simulink model "es2_catena_aperta_1"  (R2014a)
settings: Solver=ode45  StartTime=0.0  StopTime=10.0  RelTol=1e-3
libraries: cstblocks x3
settings Model: Creator=HP  LastModifiedBy=HP

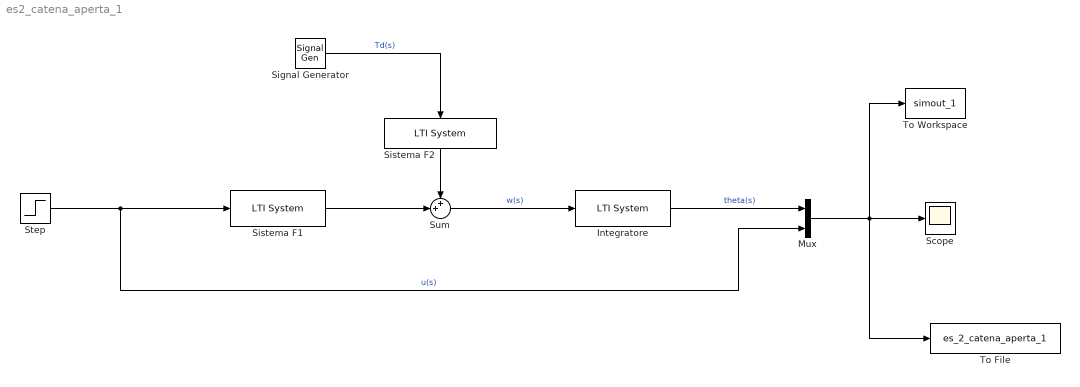
== system es2_catena_aperta_1 ==
  Integratore : cstblocks/LTI System  sys=I  IC=[]
  Mux : Mux  Inputs=2
  Scope : Scope
  Signal Generator : SignalGenerator  WaveForm=square  Amplitude=0  Units=rad/sec
  Sistema F1 : cstblocks/LTI System  sys=F1  IC=[]
  Sistema F2 : cstblocks/LTI System  sys=F2  IC=[]
  Step : Step  Time=0  SampleTime=0
  Sum : Sum  Inputs=++|
  To File : ToFile  Filename=es_2_catena_aperta_1  MatrixName=output_1  SaveFormat=Timeseries
  To Workspace : ToWorkspace  VariableName=simout_1  SaveFormat=Timeseries  SampleTime=-1
  wires:
  Step/1 -> Mux/2, Sistema F1/1  "u(s)"
  Sistema F1/1 -> Sum/2
  Sistema F2/1 -> Sum/1
  Signal Generator/1 -> Sistema F2/1  "Td(s)"
  Sum/1 -> Integratore/1  "w(s)"
  Integratore/1 -> Mux/1  "theta(s)"
  Mux/1 -> To File/1, Scope/1, To Workspace/1
